simulink model "simulink_experiment_debug_type1"  (R2016b)
settings: Solver=ode4  StartTime=0.0  StopTime=10  FixedStep=0.002  RelTol=1e-3  AbsTol=1e-6  EnableMultiTasking=on
undefined symbols (not defined in the file): HIL, qc_get_step_size
libraries: quarc_library x4, simulink_extras x2
settings Model: SimulationMode=external  ExtModeTrigDuration=50000  Creator=MLevis  LastModifiedBy=ee222-aat
settings SolverCC: PositivePriorityOrder=on
settings DataIOCC: MaxDataPoints=9000  SaveFormat=Array  SignalLoggingSaveFormat=ModelDataLogs
settings OptimizationCC: BlockReduction=off  BooleanDataType=off  OptimizeBlockIOStorage=off  BufferReuse=off  GlobalBufferReuse=off  ExpressionFolding=off  ExpressionDepthLimit=2147483647  LocalBlockOutputs=off  InitFltsAndDblsToZero=on
settings DebuggingCC: SaveWithParameterizedLinksMsg=none  UnderspecifiedInitializationDetection=Classic  MergeDetectMultiDrivingBlocksExec=none  SignalResolutionControl=TryResolveAllWithWarning  MultiTaskDSMMsg=warning  MultiTaskCondExecSysMsg=none  FcnCallInpInsideContextMsg=warning  StateNameClashWarn=warning  SFUnexpectedBacktrackingDiag=warning  SFNoUnconditionalDefaultTransitionDiag=warning  SFExecutionAtInitializationDiag=none
settings HardwareCC: TargetHWDeviceType=32-bit Generic
settings ModelReferenceCC: PropagateSignalLabelsOutOfModel=off
settings RTWCC: SystemTargetFile=quarc_win64.tlc  TemplateMakefile=quarc_default_tmf  Description=QUARC Win64 Target  BuildConfiguration=Faster Runs
settings STFCustomTargetCC: TargetPreCompLibLocation=C:\PROGRA~3\QUARC\lib\2016b\win64\release  ConcurrentExecutionCompliant=on  SystemTargetFile=quarc_win64.tlc
settings GRTTargetCC: TargetPreCompLibLocation=C:\PROGRA~3\QUARC\lib\2016b\win64\release  TargetLangStandard=C89/C90 (ANSI)  ParMdlRefBuildCompliant=off  CompOptLevelCompliant=off  CombineOutputUpdateFcns=off  MatFileLogging=off  CPPClassGenCompliant=off  GRTInterface=on  UseToolchainInfoCompliant=off  ExtMode=on  ExtModeMexFile=quarc_comm
settings ConfigComp: CovMetricSettings=dw  CovSaveCumulativeToWorkspaceVar=on  CovSaveSingleToWorkspaceVar=on  CovExternalEMLEnable=off

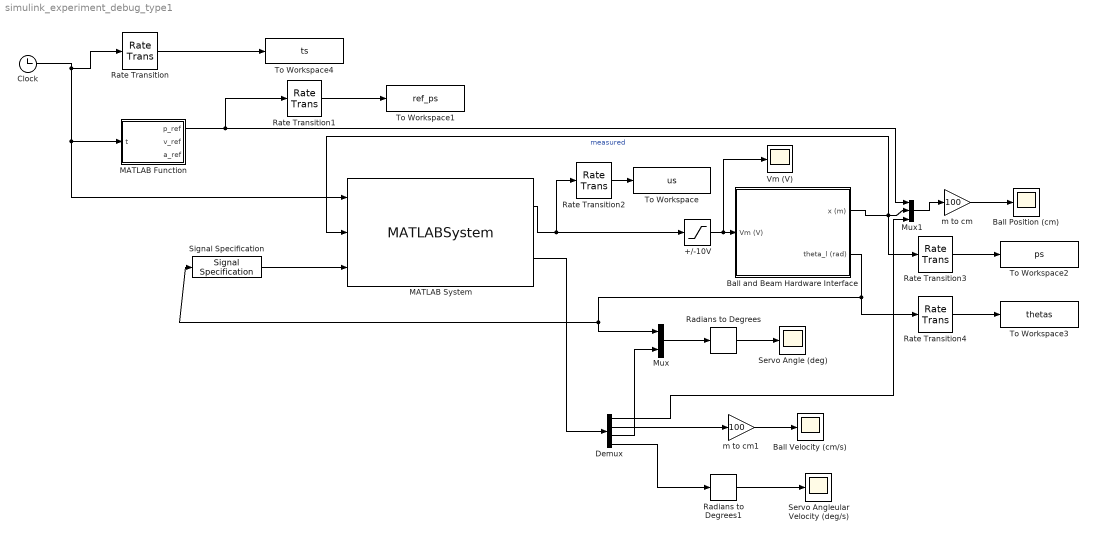
== system simulink_experiment_debug_type1 ==
  +/-10V : Saturate  UpperLimit=10  LowerLimit=-10
  Ball Position (cm) : Scope
  Ball Velocity (cm/s) : Scope
  Ball and Beam Hardware Interface : Subsystem
  Clock : Clock
  Demux : Demux
  MATLAB Function : MATLAB Function  TreatAsAtomicUnit=on
  MATLAB System : MATLABSystem  System=studentControllerInterface  SimulateUsing=Code generation
      mask Type: studentControllerInterface
      mask Display:
      | disp('studentControllerInterface');
      | port_label('input',1,'t');
      | port_label('input',2,'p_ball_obs');
      | port_label('input',3,'theta_obs');
      | port_label('output',1,'V_servo');
      | port_label('output',2,'ukf_state');
  Mux : Mux  Inputs=2
  Mux1 : Mux  Inputs=3
  Radians to Degrees : simulink_extras/Transformations/Radians to Degrees
  Radians to Degrees1 : simulink_extras/Transformations/Radians to Degrees
  Rate Transition{,1..4} (5 alike) : RateTransition  OutPortSampleTimeOpt=Inherit
  Servo Angle (deg) : Scope
  Servo Angleular Velocity (deg/s) : Scope
  Signal Specification : SignalSpecification  OutDataTypeStr=double
  To Workspace : ToWorkspace  VariableName=us  SampleTime=0.01
      settings: Save2DSignal=2-D array (concatenate along first dimension)
  To Workspace1 : ToWorkspace  VariableName=ref_ps  SampleTime=0.01
      settings: Save2DSignal=2-D array (concatenate along first dimension)
  To Workspace2 : ToWorkspace  VariableName=ps  SampleTime=0.01
      settings: Save2DSignal=2-D array (concatenate along first dimension)
  To Workspace3 : ToWorkspace  VariableName=thetas  SampleTime=0.01
      settings: Save2DSignal=2-D array (concatenate along first dimension)
  To Workspace4 : ToWorkspace  VariableName=ts  SampleTime=0.01
      settings: Save2DSignal=2-D array (concatenate along first dimension)
  Vm (V) : Scope
  m to cm : Gain  Gain=100
  m to cm1 : Gain  Gain=100
  wires:
  Radians to Degrees/1 -> Servo Angle (deg)/1
  Mux1/1 -> m to cm/1
  m to cm/1 -> Ball Position (cm)/1
  Ball and Beam Hardware Interface/1(x (m)) -> Rate Transition3/1, MATLAB System/2, Mux1/2  "measured"
  +/-10V/1 -> Vm (V)/1, Ball and Beam Hardware Interface/1(Vm (V))
  MATLAB Function/1(p_ref) -> Rate Transition1/1, Mux1/1
  Ball and Beam Hardware Interface/2(theta_l (rad)) -> Rate Transition4/1, Mux/1, Signal Specification/1
  Clock/1 -> Rate Transition/1, MATLAB Function/1(t), MATLAB System/1
  MATLAB System/1 -> Rate Transition2/1, +/-10V/1
  Signal Specification/1 -> MATLAB System/3
  Rate Transition/1 -> To Workspace4/1
  Rate Transition1/1 -> To Workspace1/1
  Rate Transition2/1 -> To Workspace/1
  Rate Transition4/1 -> To Workspace3/1
  Rate Transition3/1 -> To Workspace2/1
  MATLAB System/2 -> Demux/1
  Radians to Degrees1/1 -> Servo Angleular Velocity (deg/s)/1
  Demux/4 -> Radians to Degrees1/1
  m to cm1/1 -> Ball Velocity (cm/s)/1
  Demux/2 -> m to cm1/1
  Demux/1 -> Mux1/3
  Mux/1 -> Radians to Degrees/1
  Demux/3 -> Mux/2

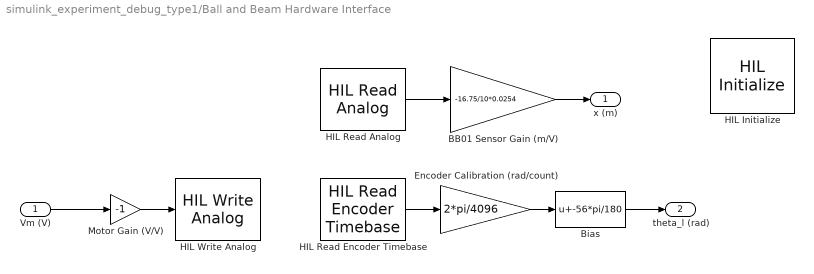
== system simulink_experiment_debug_type1/Ball and Beam Hardware Interface ==
  Vm (V) : Inport
  BB01 Sensor Gain (m/V) : Gain  Gain=-16.75/10*0.0254
  Bias : Bias  Bias=-56*pi/180
  Encoder Calibration (rad/count) : Gain  Gain=2*pi/4096  SaturateOnIntegerOverflow=on  OutDataTypeStr=Inherit: Same as input  ParamDataTypeStr=Inherit: Same as input
  HIL Initialize : quarc_library/Data Acquisition/Generic/Configuration/HIL Initialize  object_name=HIL-1  board_type=q2_usb  board_number=0  board_options=d0=digital;d1=digital;led=auto;update_rate=normal  exclusive=off  active=off  hardware_clocks=[0:2]  clock_modes=[]  initial_clock_frequencies=[]  set_clock_params_at_start=off  set_clock_params_at_switch_in=off  set_clock_frequencies_at_start=off  set_clock_frequencies_at_switch_in=off  analog_input_channels=[0:1]  analog_input_configurations=[]  analog_input_maximums=10  analog_input_minimums=-10  set_analog_input_params_at_start=on  set_analog_input_params_at_switch_in=off  analog_output_channels=[0:1]  analog_output_maximums=10  analog_output_minimums=-10  initial_analog_outputs=[0]  final_analog_outputs=[0]  watchdog_analog_outputs=0  set_analog_output_params_at_start=on  set_analog_output_params_at_switch_in=off  set_analog_outputs_at_start=on  set_analog_outputs_at_switch_in=off  set_analog_outputs_at_terminate=on  set_analog_outputs_at_switch_out=off  set_analog_outputs_on_watchdog=off  digital_input_channels=[]  digital_output_channels=[0:7]  digital_output_configuration=[]  initial_digital_outputs=[0]  final_digital_outputs=[0]  watchdog_digital_outputs=[0]  set_digital_output_params_at_start=off  set_digital_output_params_at_switch_in=off  set_digital_outputs_at_start=on  set_digital_outputs_at_switch_in=off  set_digital_outputs_at_terminate=on  set_digital_outputs_at_switch_out=off  set_digital_outputs_on_watchdog=off  encoder_channels=[0:1]  quadrature=[4]  encoder_filter_frequency=[]  initial_encoder_counts=[0]  set_encoder_params_at_start=on  set_encoder_params_at_switch_in=off  set_encoder_counts_at_start=on  set_encoder_counts_at_switch_in=off  pwm_channels=[]  pwm_modes=[0]  pwm_frequency=1/0.020  pwm_configuration=[]  pwm_alignment=[]  pwm_polarity=[]  pwm_leading_deadband=[]  pwm_trailing_deadband=[]  initial_pwm_outputs=[0]  final_pwm_outputs=[0]  watchdog_pwm_outputs=[0]  set_pwm_params_at_start=on  set_pwm_params_at_switch_in=off  set_pwm_outputs_at_start=on  set_pwm_outputs_at_switch_in=off  set_pwm_outputs_at_terminate=on  set_pwm_outputs_at_switch_out=off  set_pwm_outputs_on_watchdog=off  other_output_channels=[]  initial_other_outputs=[]  final_other_outputs=[]  watchdog_other_outputs=[]  set_other_outputs_at_start=off  set_other_outputs_at_switch_in=off  set_other_outputs_at_terminate=off  set_other_outputs_at_switch_out=off  set_other_outputs_on_watchdog=off
  HIL Read Analog : quarc_library/Data Acquisition/Generic/Immediate I//O/HIL Read Analog  object_name=HIL-1  channels=[0]  sample_time=qc_get_step_size  active=on  vector_output=off
  HIL Read Encoder Timebase : quarc_library/Data Acquisition/Generic/Timebases/HIL Read Encoder Timebase  object_name=HIL-1  clock=0  channels=0  samples_in_buffer=max(ceil(1/qc_get_step_size), 1)  active=on  vector_output=off  data_type_mode=Inherit via back propagation  data_type=double
  HIL Write Analog : quarc_library/Data Acquisition/Generic/Immediate I//O/HIL Write Analog  Tag=unassigned  object_name=HIL-1  channels=0  sample_time=-1  active=off  vector_input=off
  Motor Gain (V/V) : Gain  Gain=-1
  x (m) : Outport
  theta_l (rad) : Outport  Port=2
  wires:
  HIL Read Encoder Timebase/1 -> Encoder Calibration (rad/count)/1
  Encoder Calibration (rad/count)/1 -> Bias/1
  HIL Read Analog/1 -> BB01 Sensor Gain (m/V)/1
  Vm (V)/1 -> Motor Gain (V/V)/1
  Motor Gain (V/V)/1 -> HIL Write Analog/1
  Bias/1 -> theta_l (rad)/1
  BB01 Sensor Gain (m/V)/1 -> x (m)/1

== matlab function simulink_experiment_debug_type1/MATLAB Function ==
  data: t input; p_ref output; v_ref output; a_ref output
function [p_ref, v_ref, a_ref] = fcn(t)

[p_ref, v_ref, a_ref] = get_ref_traj(t);
